simulink model "guven2"  (R2020b)
settings: Solver=VariableStepAuto  StartTime=0.0  StopTime=5.0  RelTol=1e-3
settings Model: Creator=yakup  LastModifiedBy=yakup

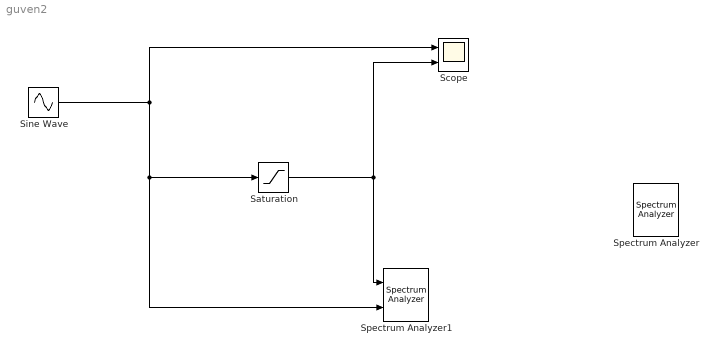
== system guven2 ==
  Saturation : Saturate  UpperLimit=1  LowerLimit=-1
  Scope : Scope  NumInputPorts=2
  Sine Wave : Sin  Amplitude=2  Frequency=200*pi  SampleTime=2*(10)^(-4)
  Spectrum Analyzer : SpectrumAnalyzer  NumInputPorts=2
  Spectrum Analyzer1 : SpectrumAnalyzer  NumInputPorts=2
  wires:
  Sine Wave/1 -> Spectrum Analyzer1/2, Saturation/1, Scope/1
  Saturation/1 -> Scope/2, Spectrum Analyzer1/1
